simulink model "passivehouse_roof_node"  (R2018b)
settings: Solver=FixedStepAuto  StartTime=0.0  StopTime=3600*24  FixedStep=5  RelTol=1e-3
values from neighbouring files (symbols this model uses):
  floorOrCeilingArea = floorOrCeilingArea*1.15    [Setup_Code_EWASP_VC.m]
undefined symbols (not defined in the file or in its folder): ceilingU, DiscIntNeverNeededParam, IsTop
settings Model: Creator=cpp14rcj  LastModifiedBy=cpp14rcj

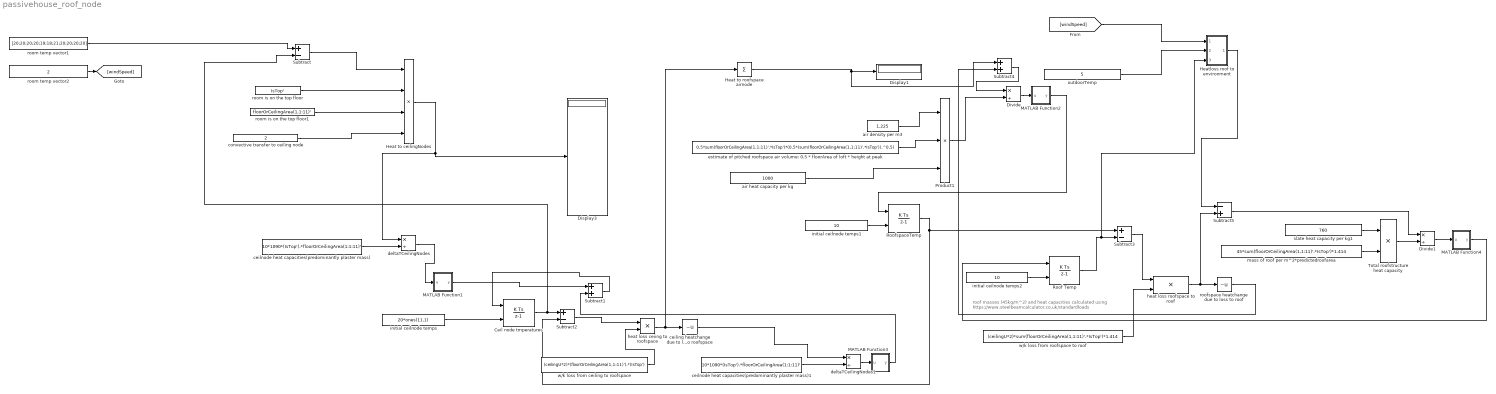
== system passivehouse_roof_node ==
  note: roof masses (45kg/m^2) and heat capacities calculated
      | using https://www.steelbeamcalculator.co.uk/standardloads
  Ceil node tmperatures : DiscreteIntegrator  InitialConditionSource=external  InitialCondition=20  SampleTime=-1  ICPrevOutput=DiscIntNeverNeededParam  ICPrevScaledInput=DiscIntNeverNeededParam
  Display1 : Display
  Display3 : Display
  Divide : Product  Inputs=*/
  Divide1 : Product  Inputs=*/
  Heat to ceilingNodes : Product  Inputs=4
  Heat to roofspace airnode : Sum  Inputs=+
  Heatloss roof to environment : Subsystem
  MATLAB Function1 : MATLAB Function  TreatAsAtomicUnit=on
  MATLAB Function2 : MATLAB Function  TreatAsAtomicUnit=on
  MATLAB Function3 : MATLAB Function  TreatAsAtomicUnit=on
  MATLAB Function4 : MATLAB Function  TreatAsAtomicUnit=on
  Product1 : Product  Inputs=3
  "Roof Temp " : DiscreteIntegrator  InitialConditionSource=external  InitialCondition=20  SampleTime=-1  ICPrevOutput=DiscIntNeverNeededParam  ICPrevScaledInput=DiscIntNeverNeededParam
  "RoofspaceTemp " : DiscreteIntegrator  InitialConditionSource=external  InitialCondition=20  SampleTime=-1  ICPrevOutput=DiscIntNeverNeededParam  ICPrevScaledInput=DiscIntNeverNeededParam
  Subtract : Sum  Inputs=+-
  Subtract1 : Sum
  Subtract2 : Sum  Inputs=+-
  Subtract3 : Sum  Inputs=+-
  Subtract4 : Sum  Inputs=2
  Subtract5 : Sum  Inputs=-+
  Total roofstructure heat capacity : Product
  air density per m3 : Constant  Value=1.225
  air heat capacity per kg : Constant  Value=1000
  ceiling heatchange due to loss to roofspace : UnaryMinus
  ceilnode heat capacities(predominantly plaster mass) : Constant  Value=10*1090*(IsTop').*floorOrCeilingArea(1:1:11)'
  ceilnode heat capacities(predominantly plaster mass)1 : Constant  Value=10*1090*(IsTop').*floorOrCeilingArea(1:1:11)'
  convective transfer to ceiling node : Constant  Value=2
  deltaTCeilingNodes : Product  Inputs=*/
  deltaTCeilingNodes1 : Product  Inputs=*/
  estimate of pitched roofspace air volume: 0.5 * floorArea of loft * height at peak : Constant  Value=0.5*sum(floorOrCeilingArea(1,1:11)'.*IsTop')*(0.5*(sum(floorOrCeilingArea(1,1:11)'.*IsTop')).^0.5)
  heat loss ceiing to roofspace : Product
  heat loss roofspace to roof : Product
  initial ceilnode temps : Constant  Value=20*ones(11,1)
  initial ceilnode temps1 : Constant  Value=10
  initial ceilnode temps2 : Constant  Value=10
  mass of roof per m^2*predictedroofarea : Constant  Value=45*sum(floorOrCeilingArea(1,1:11)'.*IsTop')*1.414
  outdoorTemp : Constant  Value=5
  roofspace heatchange due to loss to roof : UnaryMinus
  room is on the top floor : Constant  Value=IsTop'
  room is on the top floor1 : Constant  Value=floorOrCeilingArea(1,1:11)'
  room temp vector1 : Constant  Value=[20;20;20;20;19;18;21;20;20;20;20]
  room temp vector2 : Constant  Value=2
  slate heat capacity per kg1 : Constant  Value=760
  w/k loss from ceiling to roofspace : Constant  Value=(ceilingU*2)*(floorOrCeilingArea(1,1:11)').*(IsTop')
  w/k loss from roofspace to roof : Constant  Value=(ceilingU*2)*sum(floorOrCeilingArea(1,1:11)'.*IsTop')*1.414
  wires:
  room temp vector1/1 -> Subtract/1
  room is on the top floor/1 -> Heat to ceilingNodes/2
  room is on the top floor1/1 -> Heat to ceilingNodes/3
  convective transfer to ceiling node/1 -> Heat to ceilingNodes/4
  Heat to roofspace airnode/1 -> Subtract4/1, Display1/1
  Subtract/1 -> Heat to ceilingNodes/1
  estimate of pitched roofspace air volume: 0.5 * floorArea of loft * height at peak/1 -> Product1/2
  air heat capacity per kg/1 -> Product1/3
  air density per m3/1 -> Product1/1
  Product1/1 -> Divide/2
  MATLAB Function2/1(y) -> "RoofspaceTemp "/1
  initial ceilnode temps/1 -> Ceil node tmperatures/2
  ceilnode heat capacities(predominantly plaster mass)/1 -> deltaTCeilingNodes/2
  Heat to ceilingNodes/1 -> Display3/1, deltaTCeilingNodes/1
  w/k loss from ceiling to roofspace/1 -> heat loss ceiing to roofspace/2
  ceiling heatchange due to loss to roofspace/1 -> deltaTCeilingNodes1/1
  Ceil node tmperatures/1 -> Subtract/2, Subtract2/1
  initial ceilnode temps1/1 -> "RoofspaceTemp "/2
  "RoofspaceTemp "/1 -> Subtract2/2, Subtract3/1
  Subtract2/1 -> heat loss ceiing to roofspace/1
  heat loss ceiing to roofspace/1 -> Heat to roofspace airnode/1, ceiling heatchange due to loss to roofspace/1
  Subtract1/1 -> Ceil node tmperatures/1
  MATLAB Function3/1(y) -> Subtract1/2
  slate heat capacity per kg1/1 -> Total roofstructure heat capacity/1
  mass of roof per m^2*predictedroofarea/1 -> Total roofstructure heat capacity/2
  initial ceilnode temps2/1 -> "Roof Temp "/2
  "Roof Temp "/1 -> Heatloss roof to environment/3(In3), Subtract3/2
  Subtract3/1 -> heat loss roofspace to roof/1
  w/k loss from roofspace to roof/1 -> heat loss roofspace to roof/2
  roofspace heatchange due to loss to roof/1 -> Subtract4/2
  Subtract4/1 -> Divide/1
  heat loss roofspace to roof/1 -> Subtract5/2, roofspace heatchange due to loss to roof/1
  [windSpeed] -> Heatloss roof to environment/1(In1)
  outdoorTemp/1 -> Heatloss roof to environment/2(In2)
  Heatloss roof to environment/1(Out1) -> Subtract5/1
  Total roofstructure heat capacity/1 -> Divide1/2
  Subtract5/1 -> Divide1/1
  MATLAB Function4/1(y) -> "Roof Temp "/1
  deltaTCeilingNodes/1 -> MATLAB Function1/1(u)
  MATLAB Function1/1(y) -> Subtract1/1
  ceilnode heat capacities(predominantly plaster mass)1/1 -> deltaTCeilingNodes1/2
  deltaTCeilingNodes1/1 -> MATLAB Function3/1(u)
  Divide/1 -> MATLAB Function2/1(u)
  Divide1/1 -> MATLAB Function4/1(u)
  room temp vector2/1 -> [windSpeed]

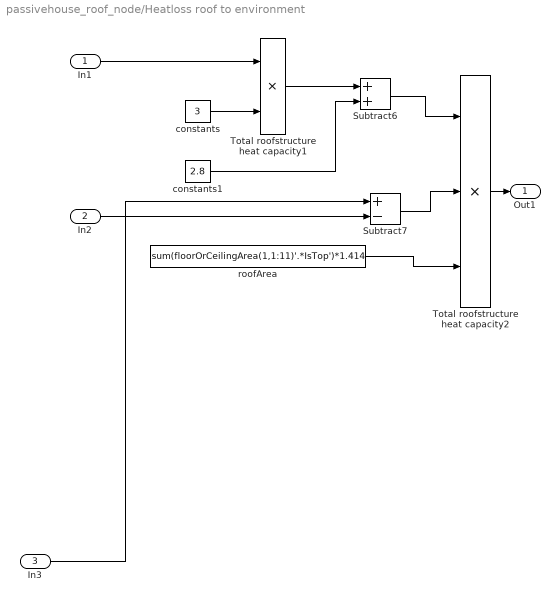
== system passivehouse_roof_node/Heatloss roof to environment ==
  In1 : Inport
  In2 : Inport  Port=2
  In3 : Inport  Port=3
  Subtract6 : Sum  Inputs=2
  Subtract7 : Sum  Inputs=+-
  Total roofstructure heat capacity1 : Product
  Total roofstructure heat capacity2 : Product  Inputs=3
  constants : Constant  Value=3
  constants1 : Constant  Value=2.8
  roofArea : Constant  Value=sum(floorOrCeilingArea(1,1:11)'.*IsTop')*1.414
  Out1 : Outport
  wires:
  Total roofstructure heat capacity2/1 -> Out1/1
  In1/1 -> Total roofstructure heat capacity1/1
  Subtract7/1 -> Total roofstructure heat capacity2/2
  constants/1 -> Total roofstructure heat capacity1/2
  Total roofstructure heat capacity1/1 -> Subtract6/1
  roofArea/1 -> Total roofstructure heat capacity2/3
  In2/1 -> Subtract7/2
  Subtract6/1 -> Total roofstructure heat capacity2/1
  constants1/1 -> Subtract6/2
  In3/1 -> Subtract7/1

== matlab function passivehouse_roof_node/MATLAB Function1 ==
  data: u input; y output
function y = fcn(u)

u(isnan(u))=0;
u(isinf(u))=0;
y=u;

== matlab function passivehouse_roof_node/MATLAB Function2 ==
  data: u input; y output
function y = fcn(u)

u(isnan(u))=0;
u(isinf(u))=0;
y=u;

== matlab function passivehouse_roof_node/MATLAB Function3 ==
  data: u input; y output
function y = fcn(u)

u(isnan(u))=0;
u(isinf(u))=0;
y=u;

== matlab function passivehouse_roof_node/MATLAB Function4 ==
  data: u input; y output
function y = fcn(u)

u(isnan(u))=0;
u(isinf(u))=0;
y=u;
